simulink model "gtm_designFS"  (Simulink 8.0)
settings: Solver=ode3  SolverMode=SingleTasking  StartTime=0.0  StopTime=50  FixedStep=Timestep  MaxStep=0.1  MinStep=0.005  RelTol=1e-5
StopFcn:
  | MWSout=grabmws(bdroot);
  | MWSout.lastrun=datestr(now);
model workspace: external: MATLAB Code tmpfile_simWS.mat (data not in the file)
undefined symbols (not defined in the file): Aero, b, bias, INU_pos, LinearizeModeOn, runway_alt, sgn, sigbuilder_block, sldvsubsys, StatesInp, symmetric_aero_on, TrimModeOn
libraries: NoiseModel_lib x28, simulink x9, GTM_FS_aerolib x3, engine_GTM_FS_lib x2, Glenn_simp2_engine_lib x2, sensors_T2_lib x2, sldvlib x2, acparams_lib x1, auxvars_lib x1, eomlib x1, actuator_FS_lib x1, Coefficient_Evaluation_lib x1
(part 1 of 3)
CloseFcn:
  | rtwprivate ssgensfun ModelCloseRequest gtm_design
settings Model: Creator=cox  LastModifiedBy=s37176  RecordCoverage=on  CovPath=NavGuidControl/Controls/Altitude Control  CovMetricSettings=dcmtrzoiw  CovHTMLOptions=-sRT=1 -aTS=1 -bRG=1 -bTC=1 -hTR=0 -nFC=0 -scm=1 -bcm=1 -xEv=0  CovModelRefEnable=all  CovExternalEMLEnable=on  ExtModeAutoUpdateStatusClock=off
settings DataIOCC: MaxDataPoints=50000  SaveFormat=Structure  SignalLoggingSaveFormat=ModelDataLogs  SaveOutput=off  SignalLogging=off
settings OptimizationCC: BooleanDataType=off  InitFltsAndDblsToZero=on
settings DebuggingCC: ConsistencyChecking=warning  SignalInfNanChecking=error  SignalRangeChecking=warning  WriteAfterWriteMsg=EnableAllAsError  SaveWithParameterizedLinksMsg=none  SignalResolutionControl=TryResolveAllWithWarning  InheritedTsInSrcMsg=none  MultiTaskDSMMsg=warning  MultiTaskCondExecSysMsg=none  CheckMatrixSingularityMsg=error  ParameterUnderflowMsg=warning  FcnCallInpInsideContextMsg=UseLocalSettings  SFcnCompatibilityMsg=warning  ModelReferenceIOMsg=warning  ModelReferenceVersionMismatchMessage=warning  ModelReferenceIOMismatchMessage=warning  ModelReferenceCSMismatchMessage=warning  InitInArrayFormatMsg=none  StrictBusMsg=Warning
settings HardwareCC: TargetHWDeviceType=32-bit Generic
settings SFSimCC: SimParseCustomCode=off
settings RTWCC: IncludeERTFirstTime=on
settings GRTTargetCC: TargetFcnLib=ansi_tfl_tmw.mat  CombineOutputUpdateFcns=off  GRTInterface=on
settings ConfigComp: Description=Design Verifier Custom Configuration Component  DVMaxTestCaseSteps=500  DVTestSuiteOptimization=CombinedObjectives (Nonlinear Extended)

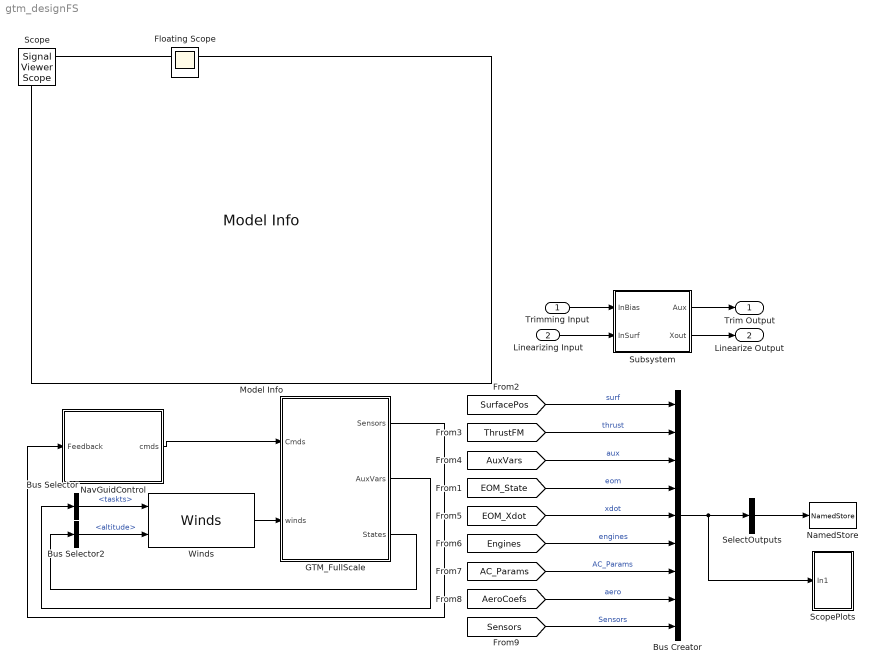
== system gtm_designFS ==
  Trimming Input : Inport  OutDataTypeStr=double  PortDimensions=4
  Linearizing Input : Inport  Port=2  OutDataTypeStr=double  PortDimensions=19
  Bus Creator : BusCreator  Inputs=9
  Bus Selector : BusSelector  OutputSignals=taskts
  Bus Selector2 : BusSelector  OutputSignals=altitude
  GTM_FullScale : Subsystem
  Model Info : simulink/Model-Wide Utilities/Model Info  InitialBlockCM=none  BlockCM=none  Frame=on  DisplayStringWithTags=|  HorizontalTextAlignment=Left  LeftAlignmentValue=0.02  SourceBlockDiagram=gtm_designFS  TagMaxNumber=20
      | Transport Class Model (TCM) Simulation or Full-Scale GTM Simulation
      | Subversion Info: %<ModelVersion>
      | Last modified by %<LastModifiedBy> on %<LastModificationDate>
      | 
      | LIMITATIONS OF SIMULATION
      | 
      | 1.  The trailing edge flap effects are not representative of a full-scale transport aircraft and, therefore,
      | any flaps-down stability and control or performance analyses would not produce any valid results.
      | 
      | 2. For Mach numbers greater than 0.6, the dyanamic response is not a valid representation of a
      | full-scale transport aircraft because the aerodynamic data is based on low-speed wind tunnel tests.
      | 
      | 3.  The Reynolds number correction is approximate.
      | 
      | 4.  The stall/post-stall dynamics are of limited fidelity due to smoothing that occurred in forming the
      | polynomial aero database.
      | 
      | 5.  There is no un-commanded roll-off response for the approach-to-stall like that of the proprietary
      | database.  The limitation is due to the lack of aerodynamic asymmetries in the polynomial model.
      | 
      | 6.  The TCM aero database does not represent the Enhanced Upset Recovery (EUR) database that
      | was developed for LaRC's Integration Flight Deck Simulator.  The TCM simulation is not valid for
      | pilot training.
      | 
      | No copyright is claimed in the United States under Title 17, U.S. Code.
      | All Other Rights Reserved.
  NamedStore : NamedStore_lib/NamedStore  Npts=inf  VarName=sout  expand=off
  NavGuidControl : Subsystem
  ScopePlots : Subsystem
  SelectOutputs : BusSelector  OutputSignals=aux.caskts,aux.alphadeg,aux.betadeg,aux.gammadeg,Sensors.InertialData.phideg,aux.gndtrackdeg,Sensors.InertialData.pbdeg,Sensors.InertialData.qbdeg,Sensors.InertialData.rbdeg  OutputAsBus=on
  Subsystem : Subsystem
  Winds : Winds_lib/Winds  WindSpeed_knots=WindSpd  WindDirection_deg=WindDir  level=None
  Trim Output : Outport  OutDataTypeStr=double  PortDimensions=9
  Linearize Output : Outport  Port=2  OutDataTypeStr=double  PortDimensions=12
  Floating Scope : Scope
      settings: Floating=on  YMin=0  YMax=7
  Scope : SignalViewerScope  IOType=viewer  RefreshTime=0.035000
  wires:
  SelectOutputs/1 -> NamedStore/1
  [SurfacePos] -> Bus Creator/1  "surf"
  [EOM_State] -> Bus Creator/4  "eom"
  [AuxVars] -> Bus Creator/3  "aux"
  [EOM_Xdot] -> Bus Creator/5  "xdot"
  [Engines] -> Bus Creator/6  "engines"
  [AC_Params] -> Bus Creator/7  "AC_Params"
  Bus Creator/1 -> SelectOutputs/1, ScopePlots/1(In1)
  NavGuidControl/1(cmds) -> GTM_FullScale/1(Cmds)
  GTM_FullScale/1(Sensors) -> NavGuidControl/1(Feedback)
  [AeroCoefs] -> Bus Creator/8  "aero"
  [Sensors] -> Bus Creator/9  "Sensors"
  Linearizing Input/1 -> Subsystem/2(InSurf)
  Subsystem/1(Aux) -> Trim Output/1
  Subsystem/2(Xout) -> Linearize Output/1
  Trimming Input/1 -> Subsystem/1(InBias)
  Bus Selector/1 -> Winds/1  "<taskts>"
  Winds/1 -> GTM_FullScale/2(winds)
  GTM_FullScale/2(AuxVars) -> Bus Selector/1
  Bus Selector2/1 -> Winds/2  "<altitude>"
  GTM_FullScale/3(States) -> Bus Selector2/1
  [ThrustFM] -> Bus Creator/2  "thrust"

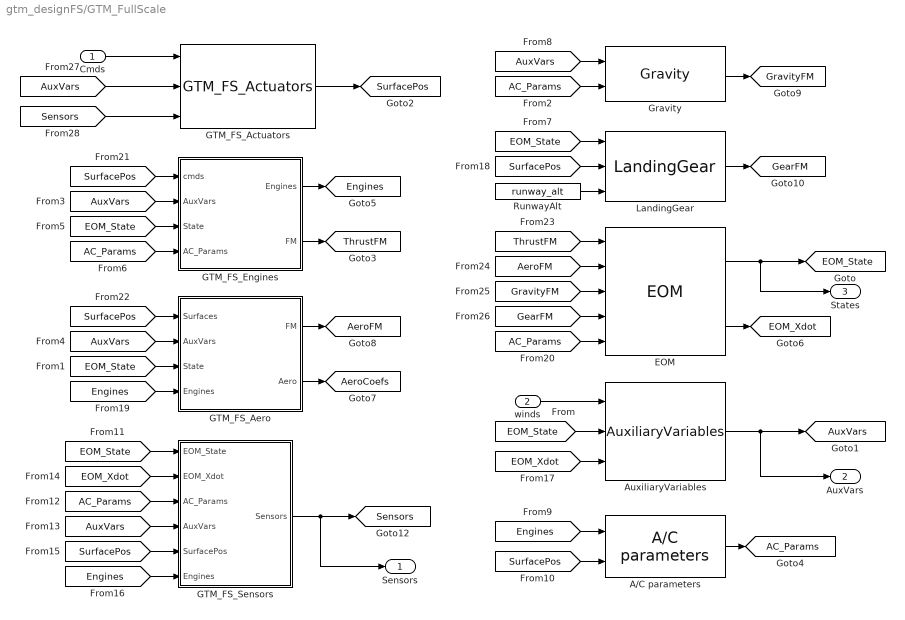
== system gtm_designFS/GTM_FullScale ==
  Cmds : Inport
  winds : Inport  Port=2  PortDimensions=6
  A/C parameters : acparams_lib/A//C parameters
  AuxiliaryVariables : auxvars_lib/AuxiliaryVariables
  EOM : eomlib/EOM
  GTM_FS_Actuators : actuator_FS_lib/GTM_FS_Actuators
  GTM_FS_Aero : Subsystem
  GTM_FS_Engines : Subsystem
  GTM_FS_Sensors : Subsystem
  Gravity : gravity_lib/Gravity
  LandingGear : landinggear_lib/LandingGear  GEAR_SPRING=25*12  zeta=0.4  NoseWheelRate=0.15
  RunwayAlt : Constant  Value=runway_alt
  Sensors : Outport
  AuxVars : Outport  Port=2
  States : Outport  Port=3
  tag scope: AC_Params=global, AeroCoefs=global, AeroFM=global, AuxVars=global, EOM_State=global, EOM_Xdot=global, Engines=global, GearFM=global, GravityFM=global, Sensors=global, SurfacePos=global, ThrustFM=global
  wires:
  GTM_FS_Actuators/1 -> [SurfacePos]
  Cmds/1 -> GTM_FS_Actuators/1
  winds/1 -> AuxiliaryVariables/1
  LandingGear/1 -> [GearFM]
  [SurfacePos] -> LandingGear/2
  [EOM_State] -> LandingGear/1
  [EOM_State] -> GTM_FS_Aero/3(State)
  AuxiliaryVariables/1 -> [AuxVars], AuxVars/1
  [AuxVars] -> GTM_FS_Aero/2(AuxVars)
  GTM_FS_Aero/1(FM) -> [AeroFM]
  GTM_FS_Engines/2(FM) -> [ThrustFM]
  EOM/1 -> [EOM_State], States/1
  [AC_Params] -> Gravity/2
  [AuxVars] -> Gravity/1
  [EOM_State] -> GTM_FS_Engines/3(State)
  [AuxVars] -> GTM_FS_Engines/2(AuxVars)
  [AC_Params] -> GTM_FS_Engines/4(AC_Params)
  A/C parameters/1 -> [AC_Params]
  [Engines] -> A/C parameters/1
  [SurfacePos] -> A/C parameters/2
  GTM_FS_Engines/1(Engines) -> [Engines]
  [EOM_Xdot] -> AuxiliaryVariables/3
  [Engines] -> GTM_FS_Aero/4(Engines)
  EOM/2 -> [EOM_Xdot]
  [SurfacePos] -> GTM_FS_Engines/1(cmds)
  RunwayAlt/1 -> LandingGear/3
  [SurfacePos] -> GTM_FS_Aero/1(Surfaces)
  GTM_FS_Aero/2(Aero) -> [AeroCoefs]
  [EOM_State] -> AuxiliaryVariables/2
  [ThrustFM] -> EOM/1
  [AeroFM] -> EOM/2
  [GravityFM] -> EOM/3
  [GearFM] -> EOM/4
  [AC_Params] -> EOM/5
  [EOM_State] -> GTM_FS_Sensors/1(EOM_State)
  [AC_Params] -> GTM_FS_Sensors/3(AC_Params)
  [SurfacePos] -> GTM_FS_Sensors/5(SurfacePos)
  [Engines] -> GTM_FS_Sensors/6(Engines)
  [EOM_Xdot] -> GTM_FS_Sensors/2(EOM_Xdot)
  [AuxVars] -> GTM_FS_Sensors/4(AuxVars)
  Gravity/1 -> [GravityFM]
  GTM_FS_Sensors/1(Sensors) -> [Sensors], Sensors/1
  [AuxVars] -> GTM_FS_Actuators/2
  [Sensors] -> GTM_FS_Actuators/3

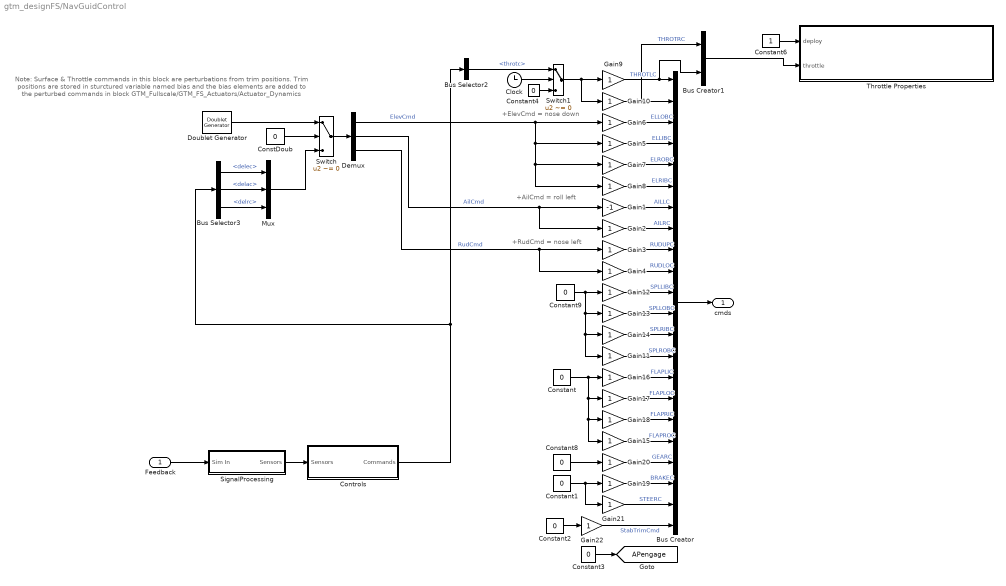
== system gtm_designFS/NavGuidControl ==
  note: +AilCmd = roll left
  note: Note: Surface & Throttle commands in this block are perturbations from
      |           trim positions.  Trim positions are stored in sturctured variable
      |          named bias and the bias elements are added to the perturbed
      |          commands in block GTM_Fullscale/GTM_FS_Actuators/Actuator_Dynamics
  note: +ElevCmd = nose down
  note: +RudCmd = nose left
  Feedback : Inport
  Bus Creator : BusCreator  Inputs=22
  Bus Creator1 : BusCreator  Inputs=2
  Bus Selector2 : BusSelector  OutputSignals=throtc
  Bus Selector3 : BusSelector  OutputSignals=delec,delac,delrc
  Clock : Clock
  ConstDoub : Constant  Value=0
  Constant{,1..4,8..9} (7 alike) : Constant  Value=0
  Constant6 : Constant
  Controls : Subsystem
  Demux : Demux  Outputs=3
  Doublet Generator : Doublet_Generator_lib/Doublet Generator  timeon=[2 22 12]  pulsewidth=[1.0 1.0 1.0]  amplitude=[0 0 0]
  Gain1 : Gain  Gain=-1  SaturateOnIntegerOverflow=on  OutDataTypeStr=Inherit: Same as input  ParamDataTypeStr=Inherit: Same as input
  Gain{2..22} (21 alike) : Gain  SaturateOnIntegerOverflow=on  OutDataTypeStr=Inherit: Same as input  ParamDataTypeStr=Inherit: Same as input
  Mux : Mux  Inputs=3
  SignalProcessing : Subsystem
  Switch : Switch  Criteria=u2 ~= 0
  Switch1 : Switch  Criteria=u2 ~= 0
  Throttle Properties : Subsystem  Tag=VerificationSubsystem  DisableCoverage=on  LoadFcn=sldvsubsys('check')  TreatAsAtomicUnit=on  SimViewingDevice=on  mask(VerificationSubsystem){}
      mask init:
      | sldvsubsys('maskInit');
      settings: CopyFcn=sldvsubsys('copy');  OpenFcn=open_system(gcb,'force');
      settings: PreSaveFcn=|
      | set_param(gcb,'SimViewingDevice','on');
      | sldvsubsys('check');
      mask Help: helpview(fullfile(docroot,'toolbox','sldv','sldv.map'),'verificationsubsystem')
      mask Display: image(imread('sldvicon_versubsys.png','BackGroundColor',[1 1 1]),'center');
  cmds : Outport
  tag scope: APengage=global
  wires:
  Constant2/1 -> Gain22/1
  Gain22/1 -> Bus Creator/22  "StabTrimCmd"
  Constant3/1 -> [APengage]
  Feedback/1 -> SignalProcessing/1(Sim In)
  Gain12/1 -> Bus Creator/11  "SPLLIBC"
  Gain13/1 -> Bus Creator/12  "SPLLOBC"
  Gain14/1 -> Bus Creator/13  "SPLRIBC"
  Gain11/1 -> Bus Creator/14  "SPLROBC"
  Gain16/1 -> Bus Creator/15  "FLAPLIC"
  Gain17/1 -> Bus Creator/16  "FLAPLOC"
  Gain18/1 -> Bus Creator/17  "FLAPRIC"
  Gain15/1 -> Bus Creator/18  "FLAPROC"
  Gain9/1 -> Bus Creator1/2, Bus Creator/1  "THROTLC"
  Gain10/1 -> Bus Creator1/1, Bus Creator/2  "THROTRC"
  Gain5/1 -> Bus Creator/4  "ELLIBC"
  Gain6/1 -> Bus Creator/3  "ELLOBC"
  Gain7/1 -> Bus Creator/5  "ELROBC"
  Gain8/1 -> Bus Creator/6  "ELRIBC"
  Gain1/1 -> Bus Creator/7  "AILLC"
  Gain2/1 -> Bus Creator/8  "AILRC"
  Gain3/1 -> Bus Creator/9  "RUDUPC"
  Gain4/1 -> Bus Creator/10  "RUDLOC"
  Switch1/1 -> Gain10/1, Gain9/1
  Constant/1 -> Gain16/1, Gain17/1, Gain18/1, Gain15/1
  Demux/2 -> Gain1/1, Gain2/1  "AilCmd"
  Demux/3 -> Gain3/1, Gain4/1  "RudCmd"
  Gain19/1 -> Bus Creator/20  "BRAKEC"
  Constant8/1 -> Gain20/1
  Constant1/1 -> Gain19/1, Gain21/1
  Demux/1 -> Gain6/1, Gain5/1, Gain7/1, Gain8/1  "ElevCmd"
  Bus Creator/1 -> cmds/1
  Gain20/1 -> Bus Creator/19  "GEARC"
  Gain21/1 -> Bus Creator/21  "STEERC"
  Doublet Generator/1 -> Switch/1
  Mux/1 -> Switch/3
  Switch/1 -> Demux/1
  ConstDoub/1 -> Switch/2
  Constant9/1 -> Gain12/1, Gain11/1, Gain14/1, Gain13/1
  Constant4/1 -> Switch1/3
  Clock/1 -> Switch1/2
  SignalProcessing/1(Sensors) -> Controls/1(Sensors)
  Bus Selector2/1 -> Switch1/1  "<throtc>"
  Controls/1(Commands) -> Bus Selector2/1, Bus Selector3/1
  Bus Selector3/1 -> Mux/1  "<delec>"
  Bus Selector3/2 -> Mux/2  "<delac>"
  Bus Selector3/3 -> Mux/3  "<delrc>"
  Bus Creator1/1 -> Throttle Properties/2(throttle)
  Constant6/1 -> Throttle Properties/1(deploy)

== system gtm_designFS/ScopePlots ==
  In1 : Inport
  Bus Selector1 : BusSelector  OutputSignals=eom.altitude,aux.caskts,aux.alphadeg,eom.theta,eom.qb,Sensors.InertialData.hdd,xdot.altitude_dot,surf.ELLOB,surf.STAB,eom.psi,eom.phi,eom.pb,eom.rb,aux.betadeg,surf.AILL,surf.AILR,surf.SPLLIB,surf.SPLRIB,surf.RUDU,engines.THROTLC,engines.THROTRC,engines.RPML,engines.RPMR,engines.EGTL,engines.EGTR,engines.fuel_burn_l,engines.fuel_burn_r,engines.ThrustL,engines.ThrustR,aux.pratio,aux.tratio
  EngineScope : Scope  NumInputPorts=8
      settings: YMin=0~1000~-1~-1~1000~1000~0~0  YMax=100~4000~1~1~30000~30000~1~1
  Gain{,1..5} (6 alike) : Gain  Gain=180/pi
  LatScope : Scope  NumInputPorts=7
      settings: YMin=0~-30~-20~-4~-20~0~-4  YMax=360~30~20~4~20~40~4  SaveName=ScopeData2
  LonScope : Scope  NumInputPorts=9
      settings: YMin=5000~100~0~0~-5~-5~-20~-20~0  YMax=12000~300~8~8~5~5~20~20~100  SaveName=ScopeData3
  Mux{1..7,9} (8 alike) : Mux  Inputs=2
  wires:
  Mux1/1 -> LatScope/3
  Mux2/1 -> LatScope/5
  Mux3/1 -> LatScope/6
  Bus Selector1/1 -> LonScope/1  "<altitude>"
  Bus Selector1/2 -> LonScope/2  "<caskts>"
  Bus Selector1/4 -> Gain/1  "<theta>"
  Bus Selector1/12 -> Gain4/1  "<pb>"
  Bus Selector1/13 -> Gain5/1  "<rb>"
  Bus Selector1/14 -> LatScope/4  "<betadeg>"
  Bus Selector1/15 -> Mux2/1  "<AILL>"
  Bus Selector1/16 -> Mux2/2  "<AILR>"
  Bus Selector1/17 -> Mux3/1  "<SPLLIB>"
  Bus Selector1/18 -> Mux3/2  "<SPLRIB>"
  Bus Selector1/19 -> LatScope/7  "<RUDU>"
  Bus Selector1/20 -> Mux4/1  "<THROTLC>"
  Bus Selector1/21 -> Mux4/2  "<THROTRC>"
  Mux4/1 -> EngineScope/1, LonScope/9
  Bus Selector1/22 -> Mux5/1  "<RPML>"
  Bus Selector1/23 -> Mux5/2  "<RPMR>"
  Mux5/1 -> EngineScope/2
  Bus Selector1/24 -> Mux6/1  "<EGTL>"
  Bus Selector1/25 -> Mux6/2  "<EGTR>"
  Bus Selector1/26 -> Mux7/1  "<fuel_burn_l>"
  Bus Selector1/27 -> Mux7/2  "<fuel_burn_r>"
  Mux6/1 -> EngineScope/3
  Mux7/1 -> EngineScope/4
  Bus Selector1/3 -> LonScope/3  "<alphadeg>"
  Bus Selector1/5 -> Gain1/1  "<qb>"
  Bus Selector1/6 -> LonScope/6  "<hdd>"
  Gain/1 -> LonScope/4  "thetadeg"
  Gain2/1 -> LatScope/1  "psideg"
  Gain3/1 -> LatScope/2  "phideg"
  Gain4/1 -> Mux1/1  "pbdeg"
  Gain5/1 -> Mux1/2  "rbdeg"
  Bus Selector1/10 -> Gain2/1  "<psi>"
  Bus Selector1/11 -> Gain3/1  "<phi>"
  Bus Selector1/7 -> LonScope/7  "<altitude_dot>"
  Gain1/1 -> LonScope/5  "qbdeg"
  Bus Selector1/28 -> EngineScope/5  "<ThrustL>"
  Bus Selector1/29 -> EngineScope/6  "<ThrustR>"
  Bus Selector1/30 -> EngineScope/7  "<pratio>"
  Bus Selector1/31 -> EngineScope/8  "<tratio>"
  Mux9/1 -> LonScope/8
  Bus Selector1/8 -> Mux9/1  "<ELLOB>"
  Bus Selector1/9 -> Mux9/2  "<STAB>"
  In1/1 -> Bus Selector1/1

== system gtm_designFS/Subsystem ==
  InBias : Inport
  InSurf : Inport  Port=2
  Bus Selector : BusSelector  OutputSignals=caskts,taskts,alphadeg,betadeg,gammadeg,gndtrackdeg,Vnkts,Vekts,Vd_fps  OutputAsBus=on
  Bus to Vector : BusToVector
  Bus to Vector1 : BusToVector
  DocBlock : simulink/Model-Wide Utilities/DocBlock  DocumentType=Text
      content=|
      | Inputs and Outputs selected here have a specific ordering.
      |
      |
      |
      | Do not change this without also changing output channel ordering in associated linmodel.m and
      | trimgtm.m functions
  Aux : Outport
  Xout : Outport  Port=2
  tag scope: SurfaceBias=global, SurfaceDeltas=global
  wires:
  [AuxVars] -> Bus Selector/1  "aux"
  [EOM_State] -> Bus to Vector1/1  "eom"
  Bus Selector/1 -> Bus to Vector/1
  InSurf/1 -> [SurfaceDeltas]
  Bus to Vector/1 -> Aux/1
  Bus to Vector1/1 -> Xout/1
  InBias/1 -> [SurfaceBias]

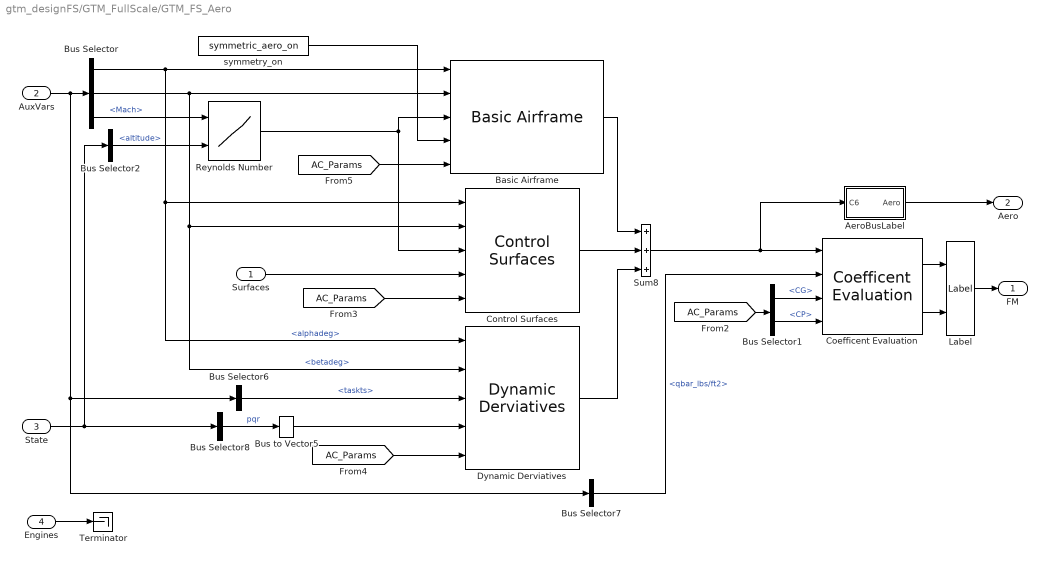
== system gtm_designFS/GTM_FullScale/GTM_FS_Aero ==
  Surfaces : Inport
  AuxVars : Inport  Port=2
  State : Inport  Port=3
  Engines : Inport  Port=4
  AeroBusLabel : Subsystem
  Basic Airframe : GTM_FS_aerolib/Basic Airframe
  Bus Selector : BusSelector  OutputSignals=alphadeg,betadeg,Mach
  Bus Selector1 : BusSelector  OutputSignals=CG,CP
  Bus Selector2 : BusSelector  OutputSignals=altitude
  Bus Selector6 : BusSelector  OutputSignals=taskts
  Bus Selector7 : BusSelector  OutputSignals=qbar_lbs/ft2
  Bus Selector8 : BusSelector  OutputSignals=pb,qb,rb  OutputAsBus=on
  Bus to Vector5 : BusToVector
  Coefficent Evaluation : Coefficient_Evaluation_lib/Coefficent Evaluation  b=b  cbar=Cbar  Sref=S
  Control Surfaces : GTM_FS_aerolib/Control Surfaces
  Dynamic Derviatives : GTM_FS_aerolib/Dynamic Derviatives
  Label : aero_lib/GTM_T2/Label
  Reynolds Number : Lookup2D  RowIndex=Aero.Reyn.mach  ColumnIndex=Aero.Reyn.alt  Table=Aero.Reyn.data
  Sum8 : Sum  Inputs=+++  SaturateOnIntegerOverflow=on  InputSameDT=on  OutDataTypeStr=Inherit: Same as first input
  Terminator : Terminator
  symmetry_on : Constant  Value=symmetric_aero_on
  FM : Outport
  Aero : Outport  Port=2
  wires:
  Reynolds Number/1 -> Control Surfaces/3, Basic Airframe/3
  symmetry_on/1 -> Basic Airframe/4
  [AC_Params] -> Basic Airframe/5
  Bus Selector2/1 -> Reynolds Number/2  "<altitude>"
  Bus Selector/3 -> Reynolds Number/1  "<Mach>"
  Surfaces/1 -> Control Surfaces/4
  [AC_Params] -> Control Surfaces/5
  [AC_Params] -> Dynamic Derviatives/5
  Bus to Vector5/1 -> Dynamic Derviatives/4
  Bus Selector6/1 -> Dynamic Derviatives/3  "<taskts>"
  Bus Selector8/1 -> Bus to Vector5/1  "pqr"
  Engines/1 -> Terminator/1
  Basic Airframe/1 -> Sum8/1
  Control Surfaces/1 -> Sum8/2
  Dynamic Derviatives/1 -> Sum8/3
  State/1 -> Bus Selector2/1, Bus Selector8/1
  Bus Selector/2 -> Basic Airframe/2, Dynamic Derviatives/2, Control Surfaces/2  "<betadeg>"
  Bus Selector/1 -> Basic Airframe/1, Dynamic Derviatives/1, Control Surfaces/1  "<alphadeg>"
  AuxVars/1 -> Bus Selector/1, Bus Selector6/1, Bus Selector7/1
  Label/1 -> FM/1
  Bus Selector7/1 -> Coefficent Evaluation/2  "<qbar_lbs/ft2>"
  Sum8/1 -> Coefficent Evaluation/1, AeroBusLabel/1(C6)
  Coefficent Evaluation/1 -> Label/1
  Coefficent Evaluation/2 -> Label/2
  Bus Selector1/1 -> Coefficent Evaluation/3  "<CG>"
  [AC_Params] -> Bus Selector1/1
  Bus Selector1/2 -> Coefficent Evaluation/4  "<CP>"
  AeroBusLabel/1(Aero) -> Aero/1

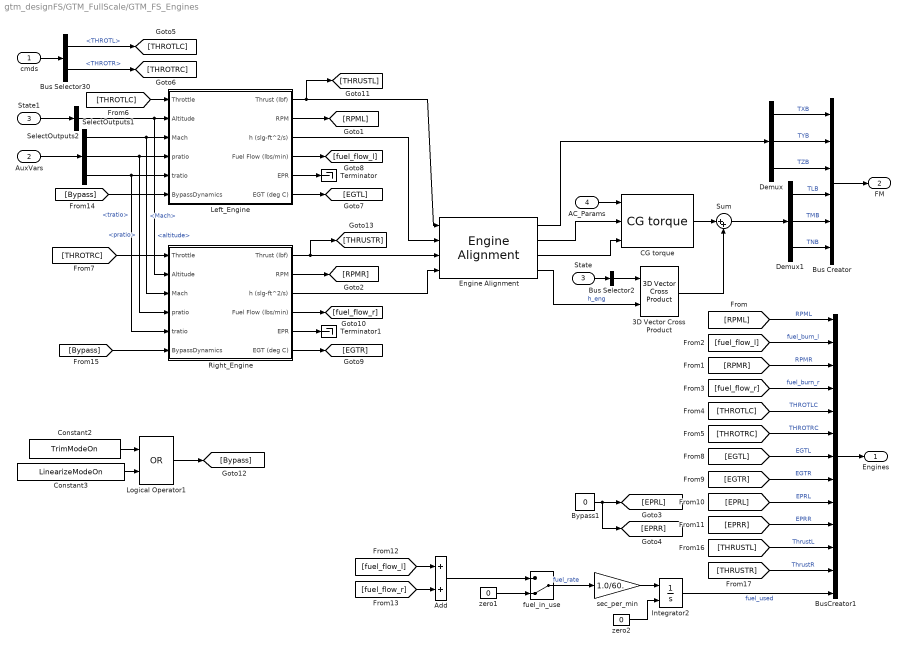
== system gtm_designFS/GTM_FullScale/GTM_FS_Engines ==
  cmds : Inport
  AuxVars : Inport  Port=2
  State : Inport  Port=3
  AC_Params : Inport  Port=4
  3D Vector Cross Product : Cross_Product_3D_lib/3D Vector Cross Product
  Add : Sum
  Bus Creator : BusCreator  Inputs=6
  Bus Selector2 : BusSelector  OutputSignals=pb,qb,rb  OutputAsBus=on
  Bus Selector30 : BusSelector  OutputSignals=THROTL,THROTR
  BusCreator1 : BusCreator  Inputs=13
  Bypass1 : Constant  Value=0
  CG torque : engine_GTM_FS_lib/GTM_FS/CG torque
  Constant2 : Constant  Value=TrimModeOn
  Constant3 : Constant  Value=LinearizeModeOn
  Demux : Demux  Outputs=3
  Demux1 : Demux  Outputs=3
  Engine Alignment : engine_GTM_FS_lib/GTM_FS/Engine Alignment
  Integrator2 : Integrator  InitialConditionSource=external
  Left_Engine : Subsystem  BlockChoice=Glenn_simp2
      settings: AttributesFormatString=%<BlockChoice>  TemplateBlock=enginelib_FS/Engine_FS  MemberBlocks=GTM_FS_Simple,Glenn_simp2
  Logical Operator1 : Logic  Operator=OR  AllPortsSameDT=off  OutDataTypeStr=boolean
  Right_Engine : Subsystem  BlockChoice=Glenn_simp2
      settings: AttributesFormatString=%<BlockChoice>  TemplateBlock=enginelib_FS/Engine_FS  MemberBlocks=GTM_FS_Simple,Glenn_simp2
  SelectOutputs1 : BusSelector  OutputSignals=Mach,pratio,tratio
  SelectOutputs2 : BusSelector  OutputSignals=altitude
  State1 : InportShadow  Port=3
  Sum : Sum  Inputs=|++
  Terminator : Terminator
  Terminator1 : Terminator
  fuel_in_use : ManualSwitch  CurrentSetting=0
  sec_per_min : Gain  Gain=1.0/60.  SaturateOnIntegerOverflow=on  OutDataTypeStr=Inherit: Same as input  ParamDataTypeStr=Inherit: Same as input
  zero1 : Constant  Value=0
  zero2 : Constant  Value=0
  Engines : Outport
  FM : Outport  Port=2  PortDimensions=6
  wires:
  cmds/1 -> Bus Selector30/1
  Demux/2 -> Bus Creator/2  "TYB"
  State/1 -> Bus Selector2/1
  Bus Selector2/1 -> 3D Vector Cross Product/1
  Demux/3 -> Bus Creator/3  "TZB"
  AuxVars/1 -> SelectOutputs1/1
  AC_Params/1 -> CG torque/1
  Bus Creator/1 -> FM/1
  Bus Selector30/1 -> [THROTLC]  "<THROTL>"
  Bus Selector30/2 -> [THROTRC]  "<THROTR>"
  [THROTLC] -> Left_Engine/1(Throttle)
  [THROTRC] -> BusCreator1/6  "THROTRC"
  [THROTLC] -> BusCreator1/5  "THROTLC"
  [fuel_flow_r] -> BusCreator1/4  "fuel_burn_r"
  [fuel_flow_l] -> BusCreator1/2  "fuel_burn_l"
  [RPMR] -> BusCreator1/3  "RPMR"
  [RPML] -> BusCreator1/1  "RPML"
  BusCreator1/1 -> Engines/1
  [EGTL] -> BusCreator1/7  "EGTL"
  [EGTR] -> BusCreator1/8  "EGTR"
  [EPRL] -> BusCreator1/9  "EPRL"
  [EPRR] -> BusCreator1/10  "EPRR"
  sec_per_min/1 -> Integrator2/1
  fuel_in_use/1 -> sec_per_min/1  "fuel_rate"
  zero2/1 -> Integrator2/2
  [fuel_flow_l] -> Add/1
  [fuel_flow_r] -> Add/2
  zero1/1 -> fuel_in_use/2
  Add/1 -> fuel_in_use/1
  Demux/1 -> Bus Creator/1  "TXB"
  Engine Alignment/4 -> 3D Vector Cross Product/2  "h_eng"
  Engine Alignment/1 -> Demux/1
  Engine Alignment/2 -> CG torque/2
  Engine Alignment/3 -> CG torque/3
  CG torque/1 -> Sum/1
  3D Vector Cross Product/1 -> Sum/2
  Demux1/1 -> Bus Creator/4  "TLB"
  Demux1/2 -> Bus Creator/5  "TMB"
  Demux1/3 -> Bus Creator/6  "TNB"
  Left_Engine/2(RPM) -> [RPML]
  Left_Engine/3(h (slg-ft^2/s)) -> Engine Alignment/2
  Left_Engine/4(Fuel Flow (lbs/min)) -> [fuel_flow_l]
  Left_Engine/6(EGT (deg C)) -> [EGTL]
  Right_Engine/2(RPM) -> [RPMR]
  Right_Engine/3(h (slg-ft^2/s)) -> Engine Alignment/4
  Right_Engine/4(Fuel Flow (lbs/min)) -> [fuel_flow_r]
  Right_Engine/6(EGT (deg C)) -> [EGTR]
  SelectOutputs1/1 -> Left_Engine/3(Mach), Right_Engine/3(Mach)  "<Mach>"
  SelectOutputs1/2 -> Left_Engine/4(pratio), Right_Engine/4(pratio)  "<pratio>"
  SelectOutputs1/3 -> Left_Engine/5(tratio), Right_Engine/5(tratio)  "<tratio>"
  [Bypass] -> Left_Engine/6(BypassDynamics)
  Left_Engine/5(EPR) -> Terminator/1
  Right_Engine/5(EPR) -> Terminator1/1
  [THROTRC] -> Right_Engine/1(Throttle)
  [Bypass] -> Right_Engine/6(BypassDynamics)
  SelectOutputs2/1 -> Left_Engine/2(Altitude), Right_Engine/2(Altitude)  "<altitude>"
  State1/1 -> SelectOutputs2/1
  Bypass1/1 -> [EPRL], [EPRR]
  Sum/1 -> Demux1/1
  Left_Engine/1(Thrust (lbf)) -> Engine Alignment/1, [THRUSTL]
  Right_Engine/1(Thrust (lbf)) -> Engine Alignment/3, [THRUSTR]
  Constant2/1 -> Logical Operator1/1
  Constant3/1 -> Logical Operator1/2
  Logical Operator1/1 -> [Bypass]
  [THRUSTL] -> BusCreator1/11  "ThrustL"
  [THRUSTR] -> BusCreator1/12  "ThrustR"
  Integrator2/1 -> BusCreator1/13  "fuel_used"

== system gtm_designFS/GTM_FullScale/GTM_FS_Sensors ==
  EOM_State : Inport
  EOM_Xdot : Inport  Port=2
  AC_Params : Inport  Port=3
  AuxVars : Inport  Port=4
  SurfacePos : Inport  Port=5
  Engines : Inport  Port=6
  AirData : Subsystem
  Bus Creator : BusCreator
  EngineData : Subsystem
  InertialData : Subsystem
  SurfaceData : Subsystem
  Sensors : Outport
  wires:
  AuxVars/1 -> AirData/1(AuxVars), InertialData/1(AuxVars)
  AirData/1(AirData) -> Bus Creator/1  "AirData"
  InertialData/1(INU) -> Bus Creator/2  "InertialData"
  SurfaceData/1(SurfPos) -> Bus Creator/3  "SurfaceData"
  EngineData/1(EngData) -> Bus Creator/4  "EngineData"
  Engines/1 -> EngineData/1(Engines)
  SurfacePos/1 -> SurfaceData/1(SurfacePos)
  EOM_Xdot/1 -> InertialData/4(EOM_Xdot)
  EOM_State/1 -> InertialData/3(EOM_State)
  AC_Params/1 -> InertialData/2(AC_Params)
  Bus Creator/1 -> Sensors/1

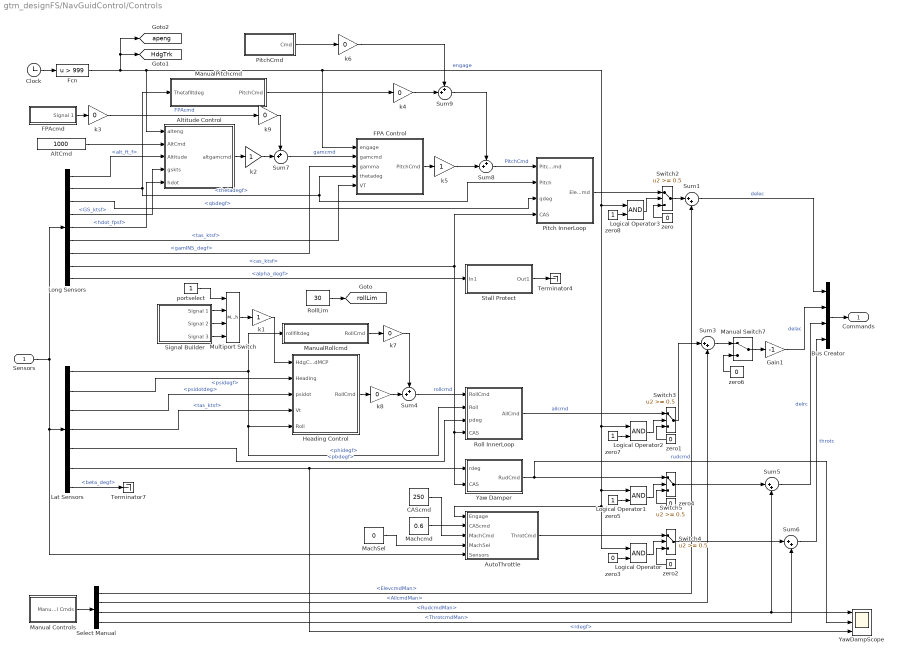
== system gtm_designFS/NavGuidControl/Controls ==
  Sensors : Inport
  AltCmd : Constant  Value=1000
  Altitude Control : Subsystem
  AutoThrottle : Subsystem
  Bus Creator : BusCreator
  CAScmd : Constant  Value=250
  Clock : Clock
  FPA Control : Subsystem
  FPAcmd : Subsystem  Tag=STV Subsys  LoadFcn=sigbuilder_block('load');  StartFcn=sigbuilder_block('start');  StopFcn=sigbuilder_block('stop');  ClipboardFcn=sigbuilder_block('clipboard');  mask(Sigbuilder block){}
      mask help: Sigbuilder GUI
      mask init:
      | if ~strcmp(get_param(bdroot(gcbh),'SimulationStatus'),'stopped') tuvar = sigbuilder_block('maskInit'); end
      settings: CopyFcn=sigbuilder_block('copy');  DeleteFcn=sigbuilder_block('delete');  ModelCloseFcn=sigbuilder_block('modelClose');  PreSaveFcn=sigbuilder_block('preSave');  PauseFcn=sigbuilder_block('pause')  ContinueFcn=sigbuilder_block('continue')  NameChangeFcn=sigbuilder_block('namechange');  OpenFcn=sigbuilder_block('open',[437.6 199.2 550.4 400 ]);  CloseFcn=sigbuilder_block('close');
      mask Display: plot(0,0,100,100,[10,10,40,40,10],[80,20,20,80,80],[40,10],[50,50], [40,27,10],[65,72,56],[40,25,25,10],[28,28,43,43]);
  Fcn : Fcn  Expr=u > 999
  Gain1 : Gain  Gain=-1  SaturateOnIntegerOverflow=on  OutDataTypeStr=Inherit: Same as input  ParamDataTypeStr=Inherit: Same as input
  Heading Control : Subsystem
  Lat Sensors : BusSelector  OutputSignals=phidegf,psidegf,EulerRates.psidotdeg,tas_ktsf,pbdegf,rdegf,beta_degf
  Logical Operator{,1..3} (4 alike) : Logic  AllPortsSameDT=off  OutDataTypeStr=boolean
  Long Sensors : BusSelector  OutputSignals=alt_ft_f,thetadegf,qbdegf,GS_ktsf,hdot_fpsf,tas_ktsf,gamINS_degf,cas_ktsf,alpha_degf
  MachSel : Constant  Value=0
  Machcmd : Constant  Value=0.6
  Manual Controls : Subsystem
  Manual Switch7 : ManualSwitch
  ManualPitchcmd : Subsystem
  ManualRollcmd : Subsystem
  Multiport Switch : MultiPortSwitch
  Pitch InnerLoop : Subsystem
  PitchCmd : Subsystem
  Roll InnerLoop : Subsystem
  RollLim : Constant  Value=30
  Select Manual : BusSelector  OutputSignals=ElevcmdMan,AilcmdMan,RudcmdMan,ThrotcmdMan
  Signal Builder : Subsystem  Tag=STV Subsys  LoadFcn=sigbuilder_block('load');  StartFcn=sigbuilder_block('start');  StopFcn=sigbuilder_block('stop');  ClipboardFcn=sigbuilder_block('clipboard');  mask(Sigbuilder block){}
      mask help: Sigbuilder GUI
      mask init:
      | if ~strcmp(get_param(bdroot(gcbh),'SimulationStatus'),'stopped') tuvar = sigbuilder_block('maskInit'); end
      settings: CopyFcn=sigbuilder_block('copy');  DeleteFcn=sigbuilder_block('delete');  ModelCloseFcn=sigbuilder_block('modelClose');  PreSaveFcn=sigbuilder_block('preSave');  PauseFcn=sigbuilder_block('pause')  ContinueFcn=sigbuilder_block('continue')  NameChangeFcn=sigbuilder_block('namechange');  OpenFcn=sigbuilder_block('open',[436.656 200.842 549.567 399.685 ]);  CloseFcn=sigbuilder_block('close');
      mask Display: plot(0,0,100,100,[10,10,40,40,10],[80,20,20,80,80],[40,10],[50,50], [40,27,10],[65,72,56],[40,25,25,10],[28,28,43,43]);
  Stall Protect : Subsystem
  Sum{1,3,5..6} (4 alike) : Sum  Inputs=|++
  Sum{4,7..9} (4 alike) : Sum  Inputs=++|
  Switch{2..5} (4 alike) : Switch  Threshold=0.5
  Terminator4 : Terminator
  Terminator7 : Terminator
  Yaw Damper : Subsystem
  YawDampScope : Scope  NumInputPorts=3
      settings: YMin=-5~-5~-5  YMax=5~5~5  SaveName=ScopeData4
  k1 : Gain
  k2 : Gain
  k{3..4,6..9} (6 alike) : Gain  Gain=0
  k5 : Gain
  portselect : Constant
  zero{,1..4,6} (6 alike) : Constant  Value=0
  zero5 : Constant
  zero7 : Constant
  zero8 : Constant
  Commands : Outport
  tag scope: HdgTrk=global, apeng=global, rollLim=global
  wires:
  Lat Sensors/6 -> YawDampScope/3, Yaw Damper/1(rdeg)  "<rdegf>"
  Lat Sensors/5 -> Roll InnerLoop/3(pdeg)  "<pbdegf>"
  Lat Sensors/4 -> Heading Control/4(Vt)  "<tas_ktsf>"
  Lat Sensors/3 -> Heading Control/3(psidot)  "<psidotdeg>"
  Lat Sensors/2 -> Heading Control/2(Heading)  "<psidegf>"
  Lat Sensors/1 -> Heading Control/5(Roll), Roll InnerLoop/2(Roll), ManualRollcmd/1(rollfiltdeg)  "<phidegf>"
  AutoThrottle/1(ThrotCmd) -> Switch4/1
  Sum6/1 -> Bus Creator/4  "throtc"
  Sum5/1 -> Bus Creator/3  "delrc"
  Gain1/1 -> Bus Creator/2  "delac"
  Sum1/1 -> Bus Creator/1  "delec"
  Bus Creator/1 -> Commands/1
  Manual Switch7/1 -> Gain1/1
  k9/1 -> Sum7/1
  k3/1 -> k9/1  "FPAcmd"
  k2/1 -> Sum7/2
  Sensors/1 -> Long Sensors/1, Lat Sensors/1, AutoThrottle/5(Sensors)
  Long Sensors/1 -> Altitude Control/3(Altitude)  "<alt_ft_f>"
  Long Sensors/2 -> Pitch InnerLoop/2(Pitch), FPA Control/4(thetadeg), ManualPitchcmd/1(Thetafiltdeg)  "<thetadegf>"
  Long Sensors/8 -> Roll InnerLoop/4(CAS), Yaw Damper/2(CAS), Pitch InnerLoop/4(CAS)  "<cas_ktsf>"
  Long Sensors/7 -> FPA Control/3(gamma)  "<gamINS_degf>"
  Long Sensors/9 -> Stall Protect/1(In1)  "<alpha_degf>"
  Clock/1 -> Fcn/1
  Manual Controls/1(Manual Cmds) -> Select Manual/1
  Select Manual/1 -> Sum1/2  "<ElevcmdMan>"
  Lat Sensors/7 -> Terminator7/1  "<beta_degf>"
  Sum3/1 -> Manual Switch7/1
  Select Manual/2 -> Sum3/2  "<AilcmdMan>"
  Switch3/1 -> Sum3/1
  Sum4/1 -> Roll InnerLoop/1(RollCmd)  "rollcmd"
  Switch5/1 -> Sum5/1
  Select Manual/3 -> Sum5/2, YawDampScope/1  "<RudcmdMan>"
  CAScmd/1 -> AutoThrottle/2(CAScmd)
  Switch4/1 -> Sum6/1
  Select Manual/4 -> Sum6/2  "<ThrotcmdMan>"
  AltCmd/1 -> Altitude Control/2(AltCmd)
  k8/1 -> Sum4/2
  zero6/1 -> Manual Switch7/2
  ManualRollcmd/1(RollCmd) -> k7/1
  Switch2/1 -> Sum1/1
  zero/1 -> Switch2/3
  Fcn/1 -> Altitude Control/1(alteng), FPA Control/1(engage), Logical Operator3/1, Logical Operator2/1, Logical Operator1/1, Logical Operator/1, AutoThrottle/1(Engage), [apeng], [HdgTrk]  "engage"
  Pitch InnerLoop/1(ElevCmd) -> Switch2/1
  Altitude Control/1(altgamcmd) -> k2/1
  Sum8/1 -> Pitch InnerLoop/1(PitchCmd)  "PitchCmd"
  ManualPitchcmd/1(PitchCmd) -> k4/1
  k5/1 -> Sum8/2
  FPA Control/1(PitchCmd) -> k5/1
  Long Sensors/5 -> Altitude Control/5(hdot)  "<hdot_fpsf>"
  Sum7/1 -> FPA Control/2(gamcmd)  "gamcmd"
  Heading Control/1(RollCmd) -> k8/1
  zero1/1 -> Switch3/3
  Roll InnerLoop/1(AilCmd) -> Switch3/1  "ailcmd"
  Logical Operator/1 -> Switch4/2
  zero3/1 -> Logical Operator/2
  zero4/1 -> Switch5/3
  Logical Operator1/1 -> Switch5/2
  zero5/1 -> Logical Operator1/2
  Yaw Damper/1(RudCmd) -> Switch5/1, YawDampScope/2  "rudcmd"
  zero7/1 -> Logical Operator2/2
  Logical Operator2/1 -> Switch3/2
  zero8/1 -> Logical Operator3/2
  Logical Operator3/1 -> Switch2/2
  FPAcmd/1(Signal 1) -> k3/1
  k7/1 -> Sum4/1
  portselect/1 -> Multiport Switch/1
  Signal Builder/1(Signal 1) -> Multiport Switch/2
  Signal Builder/2(Signal 2) -> Multiport Switch/3
  Signal Builder/3(Signal 3) -> Multiport Switch/4
  Multiport Switch/1 -> k1/1
  RollLim/1 -> [rollLim]
  k1/1 -> Heading Control/1(HdgCmdMCP)
  Stall Protect/1(Out1) -> Terminator4/1
  k4/1 -> Sum9/2
  PitchCmd/1(Cmd) -> k6/1
  Sum9/1 -> Sum8/1
  k6/1 -> Sum9/1
  Long Sensors/3 -> Pitch InnerLoop/3(qdeg)  "<qbdegf>"
  Long Sensors/4 -> Altitude Control/4(gskts)  "<GS_ktsf>"
  Long Sensors/6 -> FPA Control/5(VT)  "<tas_ktsf>"
  Machcmd/1 -> AutoThrottle/3(MachCmd)
  MachSel/1 -> AutoThrottle/4(MachSel)
  zero2/1 -> Switch4/3

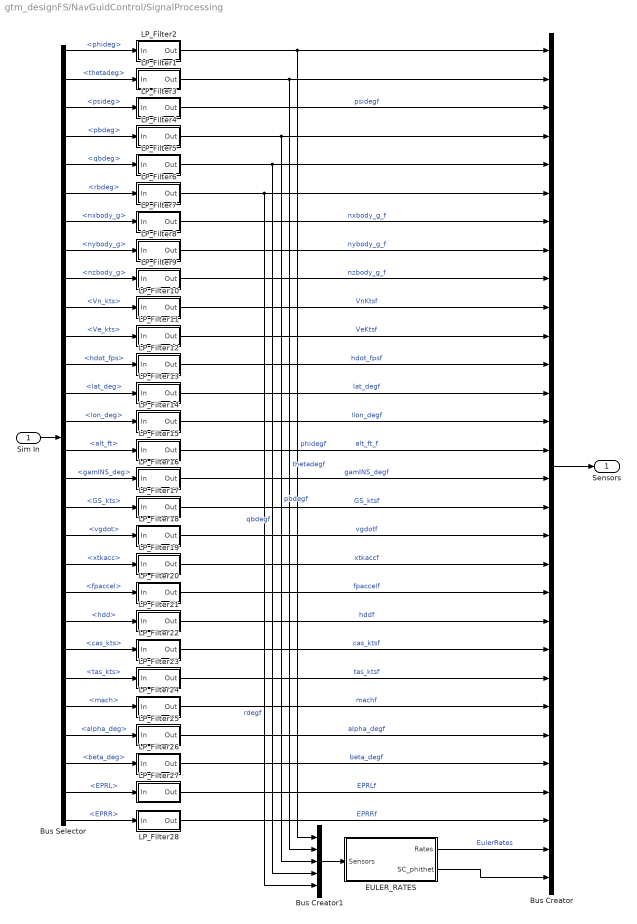
== system gtm_designFS/NavGuidControl/SignalProcessing ==
  Sim In : Inport
  Bus Creator : BusCreator  Inputs=30
  Bus Creator1 : BusCreator  Inputs=5
  Bus Selector : BusSelector  OutputSignals=InertialData.phideg,InertialData.thetadeg,InertialData.psideg,InertialData.pbdeg,InertialData.qbdeg,InertialData.rbdeg,InertialData.nxbody_g,InertialData.nybody_g,InertialData.nzbody_g,InertialData.Vn_kts,InertialData.Ve_kts,InertialData.hdot_fps,InertialData.lat_deg,InertialData.lon_deg,InertialData.alt_ft,InertialData.gamINS_deg,InertialData.GS_kts,InertialData.vgdot,InertialData.xtkacc,InertialData.fpaccel,InertialData.hdd,AirData.cas_kts,AirData.tas_kts,AirData.mach,AirData.alpha_deg,AirData.beta_deg,EngineData.EPRL,EngineData.EPRR
  EULER_RATES : Subsystem
  LP_Filter1 : Subsystem
  LP_Filter10 : Subsystem
  LP_Filter11 : Subsystem
  LP_Filter12 : Subsystem
  LP_Filter13 : Subsystem
  LP_Filter14 : Subsystem
  LP_Filter15 : Subsystem
  LP_Filter16 : Subsystem
  LP_Filter17 : Subsystem
  LP_Filter18 : Subsystem
  LP_Filter19 : Subsystem
  LP_Filter2 : Subsystem
  LP_Filter20 : Subsystem
  LP_Filter21 : Subsystem
  LP_Filter22 : Subsystem
  LP_Filter23 : Subsystem
  LP_Filter24 : Subsystem
  LP_Filter25 : Subsystem
  LP_Filter26 : Subsystem
  LP_Filter27 : Subsystem
  LP_Filter28 : Subsystem
  LP_Filter3 : Subsystem
  LP_Filter4 : Subsystem
  LP_Filter5 : Subsystem
  LP_Filter6 : Subsystem
  LP_Filter7 : Subsystem
  LP_Filter8 : Subsystem
  LP_Filter9 : Subsystem
  Sensors : Outport
  wires:
  EULER_RATES/2(SC_phithet) -> Bus Creator/30
  EULER_RATES/1(Rates) -> Bus Creator/29  "EulerRates"
  Bus Creator/1 -> Sensors/1
  Bus Creator1/1 -> EULER_RATES/1(Sensors)
  LP_Filter28/1(Out) -> Bus Creator/28  "EPRRf"
  LP_Filter27/1(Out) -> Bus Creator/27  "EPRLf"
  LP_Filter26/1(Out) -> Bus Creator/26  "beta_degf"
  LP_Filter25/1(Out) -> Bus Creator/25  "alpha_degf"
  LP_Filter24/1(Out) -> Bus Creator/24  "machf"
  LP_Filter23/1(Out) -> Bus Creator/23  "tas_ktsf"
  LP_Filter22/1(Out) -> Bus Creator/22  "cas_ktsf"
  LP_Filter21/1(Out) -> Bus Creator/21  "hddf"
  LP_Filter20/1(Out) -> Bus Creator/20  "fpaccelf"
  LP_Filter19/1(Out) -> Bus Creator/19  "xtkaccf"
  LP_Filter18/1(Out) -> Bus Creator/18  "vgdotf"
  LP_Filter17/1(Out) -> Bus Creator/17  "GS_ktsf"
  LP_Filter16/1(Out) -> Bus Creator/16  "gamINS_degf"
  LP_Filter15/1(Out) -> Bus Creator/15  "alt_ft_f"
  LP_Filter14/1(Out) -> Bus Creator/14  "llon_degf"
  LP_Filter13/1(Out) -> Bus Creator/13  "lat_degf"
  LP_Filter12/1(Out) -> Bus Creator/12  "hdot_fpsf"
  LP_Filter11/1(Out) -> Bus Creator/11  "VeKtsf"
  LP_Filter10/1(Out) -> Bus Creator/10  "VnKtsf"
  LP_Filter9/1(Out) -> Bus Creator/9  "nzbody_g_f"
  LP_Filter8/1(Out) -> Bus Creator/8  "nybody_g_f"
  LP_Filter7/1(Out) -> Bus Creator/7  "nxbody_g_f"
  LP_Filter6/1(Out) -> Bus Creator1/5, Bus Creator/6  "rdegf"
  LP_Filter5/1(Out) -> Bus Creator1/4, Bus Creator/5  "qbdegf"
  LP_Filter4/1(Out) -> Bus Creator1/3, Bus Creator/4  "pbdegf"
  LP_Filter3/1(Out) -> Bus Creator/3  "psidegf"
  LP_Filter1/1(Out) -> Bus Creator1/2, Bus Creator/2  "thetadegf"
  LP_Filter2/1(Out) -> Bus Creator1/1, Bus Creator/1  "phidegf"
  Bus Selector/28 -> LP_Filter28/1(In)  "<EPRR>"
  Bus Selector/27 -> LP_Filter27/1(In)  "<EPRL>"
  Bus Selector/26 -> LP_Filter26/1(In)  "<beta_deg>"
  Bus Selector/25 -> LP_Filter25/1(In)  "<alpha_deg>"
  Bus Selector/24 -> LP_Filter24/1(In)  "<mach>"
  Bus Selector/23 -> LP_Filter23/1(In)  "<tas_kts>"
  Bus Selector/22 -> LP_Filter22/1(In)  "<cas_kts>"
  Bus Selector/21 -> LP_Filter21/1(In)  "<hdd>"
  Bus Selector/20 -> LP_Filter20/1(In)  "<fpaccel>"
  Bus Selector/19 -> LP_Filter19/1(In)  "<xtkacc>"
  Bus Selector/18 -> LP_Filter18/1(In)  "<vgdot>"
  Bus Selector/17 -> LP_Filter17/1(In)  "<GS_kts>"
  Bus Selector/16 -> LP_Filter16/1(In)  "<gamINS_deg>"
  Bus Selector/15 -> LP_Filter15/1(In)  "<alt_ft>"
  Bus Selector/14 -> LP_Filter14/1(In)  "<lon_deg>"
  Bus Selector/13 -> LP_Filter13/1(In)  "<lat_deg>"
  Bus Selector/12 -> LP_Filter12/1(In)  "<hdot_fps>"
  Bus Selector/11 -> LP_Filter11/1(In)  "<Ve_kts>"
  Bus Selector/10 -> LP_Filter10/1(In)  "<Vn_kts>"
  Bus Selector/9 -> LP_Filter9/1(In)  "<nzbody_g>"
  Bus Selector/8 -> LP_Filter8/1(In)  "<nybody_g>"
  Bus Selector/7 -> LP_Filter7/1(In)  "<nxbody_g>"
  Bus Selector/6 -> LP_Filter6/1(In)  "<rbdeg>"
  Bus Selector/5 -> LP_Filter5/1(In)  "<qbdeg>"
  Bus Selector/4 -> LP_Filter4/1(In)  "<pbdeg>"
  Bus Selector/3 -> LP_Filter3/1(In)  "<psideg>"
  Bus Selector/2 -> LP_Filter1/1(In)  "<thetadeg>"
  Bus Selector/1 -> LP_Filter2/1(In)  "<phideg>"
  Sim In/1 -> Bus Selector/1

== system gtm_designFS/NavGuidControl/Throttle Properties ==
  note: If two thrust sensors are >0, deploy cannot be true.
  deploy : Inport
  throttle : Inport  Port=2
  Compare To Constant5 : simulink/Logic and Bit Operations/Compare To Constant  relop=>  const=-1  OutDataTypeStr=uint8  ZeroCross=off
  Compare To Constant6 : simulink/Logic and Bit Operations/Compare To Constant  relop=>  const=-1  OutDataTypeStr=uint8  ZeroCross=off
  Compare To Constant7 : simulink/Logic and Bit Operations/Compare To Constant  relop=>=  const=3  OutDataTypeStr=uint8  ZeroCross=off
  Demux2 : Demux  Outputs=[1 1]
  Implies3 : sldvlib/Verification Utilities/Implies
  Mux1 : Mux  Inputs=2
  Sum of Elements1 : Sum  Inputs=1
  throttle valid : Assertion  Enabled=on
  wires:
  Demux2/1 -> Compare To Constant5/1  "RightEngine"
  Demux2/2 -> Compare To Constant6/1  "LeftEngine"
  Sum of Elements1/1 -> Compare To Constant7/1
  Compare To Constant5/1 -> Mux1/1
  Compare To Constant6/1 -> Mux1/2
  Mux1/1 -> Sum of Elements1/1
  throttle/1 -> Demux2/1
  Compare To Constant7/1 -> Implies3/1
  deploy/1 -> Implies3/2
  Implies3/1 -> throttle valid/1

== system gtm_designFS/GTM_FullScale/GTM_FS_Aero/AeroBusLabel ==
  C6 : Inport
  Bus Creator : BusCreator  Inputs=6
  Demux : Demux  Outputs=6
  Aero : Outport
  wires:
  C6/1 -> Demux/1
  Demux/1 -> Bus Creator/1  "CX"
  Demux/2 -> Bus Creator/2  "CY"
  Demux/3 -> Bus Creator/3  "CZ"
  Demux/4 -> Bus Creator/4  "Cl"
  Demux/5 -> Bus Creator/5  "CM"
  Demux/6 -> Bus Creator/6  "CN"
  Bus Creator/1 -> Aero/1

== system gtm_designFS/GTM_FullScale/GTM_FS_Engines/Left_Engine ==
  Throttle : Inport
  Altitude : Inport  Port=2
  Mach : Inport  Port=3
  pratio : Inport  Port=4
  tratio : Inport  Port=5
  BypassDynamics : Inport  Port=6
  Glenn_simp2 : Glenn_simp2_engine_lib/Glenn_simp2
  Thrust (lbf) : Outport
  RPM : Outport  Port=2
  h (slg-ft^2/s) : Outport  Port=3
  Fuel Flow (lbs/min) : Outport  Port=4
  EPR : Outport  Port=5
  EGT (deg C) : Outport  Port=6
  wires:
  Throttle/1 -> Glenn_simp2/1
  Altitude/1 -> Glenn_simp2/2
  Mach/1 -> Glenn_simp2/3
  pratio/1 -> Glenn_simp2/4
  tratio/1 -> Glenn_simp2/5
  BypassDynamics/1 -> Glenn_simp2/6
  Glenn_simp2/1 -> Thrust (lbf)/1
  Glenn_simp2/2 -> RPM/1
  Glenn_simp2/3 -> h (slg-ft^2/s)/1
  Glenn_simp2/4 -> Fuel Flow (lbs/min)/1
  Glenn_simp2/5 -> EPR/1
  Glenn_simp2/6 -> EGT (deg C)/1

== system gtm_designFS/GTM_FullScale/GTM_FS_Engines/Right_Engine ==
  Throttle : Inport
  Altitude : Inport  Port=2
  Mach : Inport  Port=3
  pratio : Inport  Port=4
  tratio : Inport  Port=5
  BypassDynamics : Inport  Port=6
  Glenn_simp2 : Glenn_simp2_engine_lib/Glenn_simp2
  Thrust (lbf) : Outport
  RPM : Outport  Port=2
  h (slg-ft^2/s) : Outport  Port=3
  Fuel Flow (lbs/min) : Outport  Port=4
  EPR : Outport  Port=5
  EGT (deg C) : Outport  Port=6
  wires:
  Throttle/1 -> Glenn_simp2/1
  Altitude/1 -> Glenn_simp2/2
  Mach/1 -> Glenn_simp2/3
  pratio/1 -> Glenn_simp2/4
  tratio/1 -> Glenn_simp2/5
  BypassDynamics/1 -> Glenn_simp2/6
  Glenn_simp2/1 -> Thrust (lbf)/1
  Glenn_simp2/2 -> RPM/1
  Glenn_simp2/3 -> h (slg-ft^2/s)/1
  Glenn_simp2/4 -> Fuel Flow (lbs/min)/1
  Glenn_simp2/5 -> EPR/1
  Glenn_simp2/6 -> EGT (deg C)/1

== system gtm_designFS/GTM_FullScale/GTM_FS_Sensors/AirData ==
  AuxVars : Inport
  Bus Selector : BusSelector  OutputSignals=caskts,taskts,Mach,alphadeg,betadeg,qbar_lbs/ft2,qc_lbs/ft2,TAT_degC,TotalPres_lbsPerFt2,pressure_lbsPerFt2,temperature_degK,pratio,tratio
  Sensor Model1 : NoiseModel_lib/NoiseModel  noise_on=SensorNoise.On  sigma=SensorNoise.KTAS.Std  seed=278234  bias=SensorNoise.KTAS.Bias  scf=SensorNoise.KTAS.Scf
  Sensor Model2 : NoiseModel_lib/NoiseModel  noise_on=SensorNoise.On  sigma=SensorNoise.mach.Std  seed=278234  bias=SensorNoise.mach.Bias  scf=SensorNoise.mach.Scf
  Sensor Model3 : NoiseModel_lib/NoiseModel  noise_on=SensorNoise.On  sigma=SensorNoise.alpha.Std  seed=278234  bias=SensorNoise.alpha.Bias  scf=SensorNoise.alpha.Scf
  Sensor Model4 : NoiseModel_lib/NoiseModel  noise_on=SensorNoise.On  sigma=SensorNoise.beta.Std  seed=278234  bias=SensorNoise.beta.Bias  scf=SensorNoise.beta.Scf
  Sensor Model5 : NoiseModel_lib/NoiseModel  noise_on=SensorNoise.On  sigma=SensorNoise.KCAS.Std  seed=278234  bias=SensorNoise.KCAS.Bias  scf=SensorNoise.KCAS.Scf
  Sensor Model6 : NoiseModel_lib/NoiseModel  noise_on=SensorNoise.On  sigma=SensorNoise.dyn_press.Std  seed=278234  bias=SensorNoise.dyn_press.Bias  scf=SensorNoise.dyn_press.Scf
  pitot bus : BusCreator  Inputs=13
  AirData : Outport
  wires:
  Bus Selector/1 -> Sensor Model5/1  "<caskts>"
  Bus Selector/2 -> Sensor Model1/1  "<taskts>"
  Bus Selector/3 -> Sensor Model2/1  "<Mach>"
  Bus Selector/4 -> Sensor Model3/1  "<alphadeg>"
  Bus Selector/5 -> Sensor Model4/1  "<betadeg>"
  Bus Selector/6 -> Sensor Model6/1  "<qbar_lbs/ft2>"
  Sensor Model5/1 -> pitot bus/1  "cas_kts"
  Sensor Model1/1 -> pitot bus/2  "tas_kts"
  Sensor Model2/1 -> pitot bus/3  "mach"
  Sensor Model3/1 -> pitot bus/4  "alpha_deg"
  Sensor Model4/1 -> pitot bus/5  "beta_deg"
  Sensor Model6/1 -> pitot bus/6  "qbar_pf2"
  AuxVars/1 -> Bus Selector/1
  pitot bus/1 -> AirData/1
  Bus Selector/7 -> pitot bus/7  "<qc_lbs/ft2>"
  Bus Selector/8 -> pitot bus/8  "<TAT_degC>"
  Bus Selector/9 -> pitot bus/9  "<TotalPres_lbsPerFt2>"
  Bus Selector/10 -> pitot bus/10  "<pressure_lbsPerFt2>"
  Bus Selector/11 -> pitot bus/11  "<temperature_degK>"
  Bus Selector/12 -> pitot bus/12  "<pratio>"
  Bus Selector/13 -> pitot bus/13  "<tratio>"

== system gtm_designFS/GTM_FullScale/GTM_FS_Sensors/EngineData ==
  Engines : Inport
  Bus Creator : BusCreator  Inputs=6
  Bus Selector : BusSelector  OutputSignals=EPRL,EPRR,RPML,RPMR,EGTL,EGTR
  Sensor Model{1..6} (6 alike) : NoiseModel_lib/NoiseModel  noise_on=SensorNoise.On  sigma=SensorNoise.alpha.Std  seed=278234  bias=SensorNoise.alpha.Bias  scf=SensorNoise.alpha.Scf
  EngData : Outport
  wires:
  Engines/1 -> Bus Selector/1
  Bus Creator/1 -> EngData/1
  Bus Selector/1 -> Sensor Model5/1  "<EPRL>"
  Bus Selector/2 -> Sensor Model1/1  "<EPRR>"
  Bus Selector/5 -> Sensor Model4/1  "<EGTL>"
  Bus Selector/6 -> Sensor Model6/1  "<EGTR>"
  Sensor Model5/1 -> Bus Creator/1  "EPRL"
  Sensor Model1/1 -> Bus Creator/2  "EPRR"
  Sensor Model2/1 -> Bus Creator/3  "RPML"
  Sensor Model3/1 -> Bus Creator/4  "RPMR"
  Sensor Model4/1 -> Bus Creator/5  "EGTL"
  Sensor Model6/1 -> Bus Creator/6  "EGTR"
  Bus Selector/3 -> Sensor Model2/1  "<RPML>"
  Bus Selector/4 -> Sensor Model3/1  "<RPMR>"
